simulink model "SmkLim_AirMsSel"  (R2016b)
settings: configuration reference "CodeGenConfigSet" (kept outside this file)
values from neighbouring files (symbols this model uses):
  SmkLim_swtAirMs_C = Calibration.Parameter    [init_SmkLim_AirMsSel.m]    (also in init_SmkLim_AirMsSel_SIL.m = Simulink.Parameter)
settings Model: Creator=xuxingpei  LastModifiedBy=liutao
settings ConfigSetRef: SourceLocation=Base Workspace

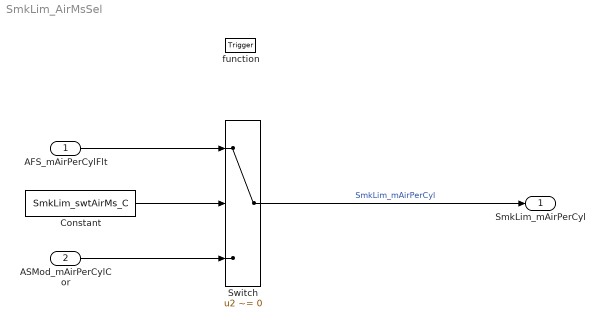
== system SmkLim_AirMsSel ==
  AFS_mAirPerCylFlt : Inport  Tag=mg/hub  Description=Filtered air mass per cylinder  OutMin=0  OutMax=16383  OutDataTypeStr=AirMass_mg_hub
  ASMod_mAirPerCylCor : Inport  Tag=mg/hub  Description=|  Port=2  OutMin=0  OutMax=16383  OutDataTypeStr=AirMass_mg_hub
      | Dynamically corrected fresh air mass per cylinder
      | upstream of the intake manifold
  function : TriggerPort  TriggerType=function-call  VariantControl=Variant
  Constant : Constant  Value=SmkLim_swtAirMs_C
  Switch : Switch  Criteria=u2 ~= 0
  SmkLim_mAirPerCyl : Outport  Tag=mg/hub  Description=Air mass for smoke limitation  OutMin=0  OutMax=16383  OutDataTypeStr=AirMass_mg_hub
  wires:
  Switch/1 -> SmkLim_mAirPerCyl/1  "SmkLim_mAirPerCyl"
  ASMod_mAirPerCylCor/1 -> Switch/3
  AFS_mAirPerCylFlt/1 -> Switch/1
  Constant/1 -> Switch/2
